simulink model "mod3_ciff_1bit"  (Simulink 7.9)
settings: Solver=ode45  StartTime=0.0  StopTime=simu.trantime  RelTol=1e-3
undefined symbols (not defined in the file): dc, Fs, mod, OSR, sinamp, sinfreq
libraries: dspsigops x3, dsparch4 x1, simulink x1, dspsrcs4 x1
settings Model: Creator=amyles  LastModifiedBy=Arnaldi Isacco
settings DataIOCC: LimitDataPoints=off  MaxDataPoints=50000
settings OptimizationCC: InlineParams=on
settings DebuggingCC: StrictBusMsg=Warning
settings ModelReferenceCC: ModelReferenceNumInstancesAllowed=Single
settings CodeAppCC: CustomSymbolStrType=$N$R$M_T
settings GRTTargetCC: CombineOutputUpdateFcns=off  GRTInterface=on

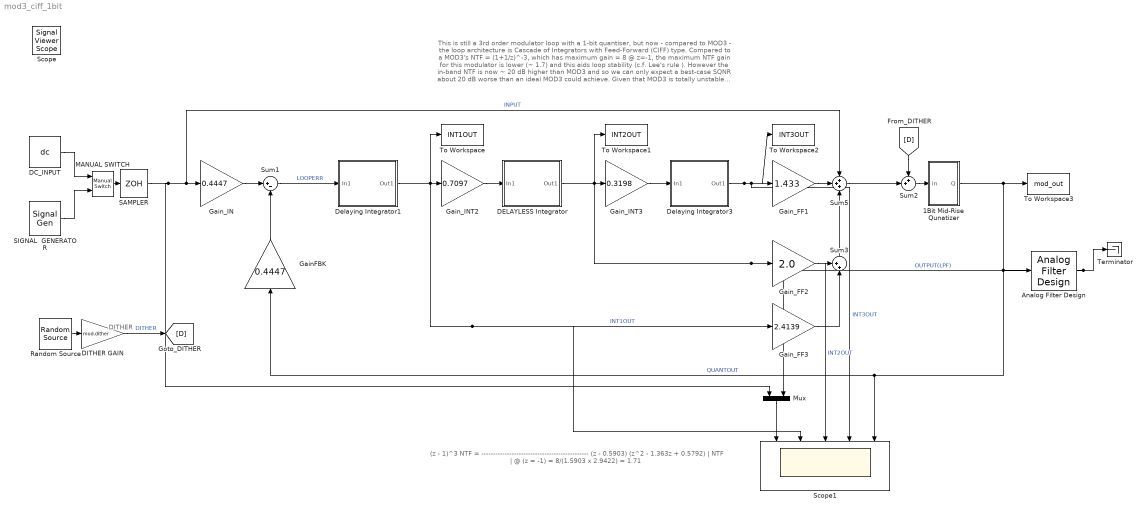
== system mod3_ciff_1bit ==
  note: This is still a 3rd order modulator loop with a 1-bit quantiser, but now - compared to MOD3 - the loop architecture is Cascade of Integrators
      | with Feed-Forward  (CIFF) type.  Compared to a MOD3's NTF = (1+1/z)^-3, which has maximum gain = 8 @ z=-1, the  maximum NTF gain for
      | this modulator is lower (~ 1.7) and this aids loop stability (c.f. Lee's rule ). However the in-band NTF is now ~ 20 dB higher than MOD3 and so
      | we can only expect a best-case SQNR about 20 dB worse than an ideal MOD3 could achieve.
      | Given that MOD3 is totally unstable and hence useless anyway, this still is a very acceptable cost to pay!
  note: (z - 1)^3
      |   NTF = ----------------------------------------------
      |            (z - 0.5903) (z^2 - 1.363z + 0.5792)
      |
      |
      | | NTF | @ (z = -1) = 8/(1.5903 x 2.9422) = 1.71
  note: DITHER
  1Bit Mid-Rise Qunatizer : Subsystem
  Analog Filter Design : dsparch4/Analog Filter Design  method=Butterworth  filttype=Lowpass  N=8  Wlo=pi*(Fs/OSR)  Whi=80  Rp=2  Rs=40
      settings: AttributesFormatString=Low-pass filter the loop output\nto illustrate intuitively how the\npulse density modulated +1/-1\noutput stream does indeed capture\nthe input signal
  DC_INPUT : Constant  Value=dc  VectorParams1D=off  OutDataTypeStr=double  SampleTime=1/Fs
  DELAYLESS Integrator : Subsystem
  DITHER GAIN : Gain  Gain=mod.dither  SampleTime=1/Fs
  Delaying Integrator1 : Subsystem
  Delaying Integrator3 : Subsystem
  GainFBK : Gain  Gain=0.4447
  Gain_FF1 : Gain  Gain=1.433
  Gain_FF2 : Gain  Gain=2.0
  Gain_FF3 : Gain  Gain=2.4139
  Gain_IN : Gain  Gain=0.4447
  Gain_INT2 : Gain  Gain=0.7097
  Gain_INT3 : Gain  Gain=0.3198
  MANUAL SWITCH : simulink/Signal Routing/Manual Switch  sw=0  action=0  varsize=off
      settings: AttributesFormatString=Double click to\nselect the desired\ninput
  Mux : Mux  Inputs=2
  Random Source : dspsrcs4/Random Source  SrcType=Uniform  NormMethod=Ziggurat  CltLength=12  MinVal=-1  MaxVal=1  MeanVal=0  VarVal=1  RepMode=Not repeatable  rawSeed=1  IsInherit=off  SampMode=Discrete  SampTime=1/Fs  SampFrame=1  DataType=Double  OutComplex=Real
  SAMPLER : ZeroOrderHold  SampleTime=1/Fs
  SIGNAL  GENERATOR : SignalGenerator  Amplitude=sinamp  Frequency=sinfreq  VectorParams1D=off
  Scope1 : Scope  NumInputPorts=5
      settings: TimeRange=2.089895171320487e-05  YMin=0.43~-0.6~-0.6~-0.3~-1.1  YMax=0.52~0.5~0.5~0.5~1.1
  Sum1 : Sum  Inputs=|+-  SampleTime=1/Fs
      settings: AttributesFormatString=Modulator input\nloop servo error (input - fbk)
  Sum2 : Sum  Inputs=++|
  Sum3 : Sum  Inputs=++|
  Sum5 : Sum  Inputs=+++
  Terminator : Terminator
  To Workspace : ToWorkspace  VariableName=INT1OUT  SampleTime=-1
  To Workspace1 : ToWorkspace  VariableName=INT2OUT  SampleTime=-1
  To Workspace2 : ToWorkspace  VariableName=INT3OUT  SampleTime=-1
  To Workspace3 : ToWorkspace  VariableName=mod_out  SampleTime=-1
      settings: AttributesFormatString=Export output to\nworkspace for\npost-processing
  Scope : SignalViewerScope  IOType=viewer  NumInputPorts=4  ZoomMode=xonly  RefreshTime=0.035000
      settings: YMin=-5~-5~-5~-5  YMax=5~5~5~5
  wires:
  Sum1/1 -> Delaying Integrator1/1(In1)  "LOOPERR"
  SAMPLER/1 -> Gain_IN/1, Sum5/1, Mux/1  "INPUT"
  1Bit Mid-Rise Qunatizer/1(Q) -> To Workspace3/1, Analog Filter Design/1, Scope1/5, GainFBK/1  "QUANTOUT"
  Delaying Integrator1/1(Out1) -> Gain_INT2/1, Gain_FF3/1, Scope1/2, To Workspace/1  "INT1OUT"
  Gain_INT2/1 -> DELAYLESS Integrator/1(In1)
  DELAYLESS Integrator/1(Out1) -> Gain_INT3/1, To Workspace1/1, Gain_FF2/1, Scope1/3  "INT2OUT"
  GainFBK/1 -> Sum1/2
  Gain_IN/1 -> Sum1/1
  Delaying Integrator3/1(Out1) -> Gain_FF1/1, To Workspace2/1, Scope1/4  "INT3OUT"
  Gain_INT3/1 -> Delaying Integrator3/1(In1)
  Gain_FF1/1 -> Sum5/2
  Gain_FF2/1 -> Sum3/1
  Sum3/1 -> Sum5/3
  Gain_FF3/1 -> Sum3/2
  Random Source/1 -> DITHER GAIN/1
  DITHER GAIN/1 -> [D]  "DITHER"
  [D] -> Sum2/1
  Sum2/1 -> 1Bit Mid-Rise Qunatizer/1(in)
  Sum5/1 -> Sum2/2
  Analog Filter Design/1 -> Terminator/1, Mux/2  "OUTPUT(LPF)"
  DC_INPUT/1 -> MANUAL SWITCH/1
  SIGNAL  GENERATOR/1 -> MANUAL SWITCH/2
  MANUAL SWITCH/1 -> SAMPLER/1
  Mux/1 -> Scope1/1

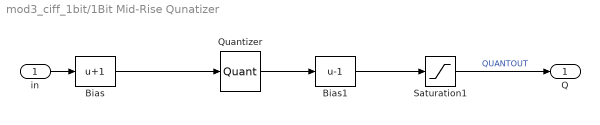
== system mod3_ciff_1bit/1Bit Mid-Rise Qunatizer ==
  in : Inport
  Bias : Bias  Bias=1
      settings: AttributesFormatString=Need offset to give\nMID-RISE quantiser
  Bias1 : Bias  Bias=-1
  Quantizer : Quantizer  QuantizationInterval=2  LinearizeAsGain=off  SampleTime=1/Fs
  Saturation1 : Saturate  UpperLimit=1  LowerLimit=-1
      settings: AttributesFormatString=Limit quantiser\noutput to +/-1
  Q : Outport
  wires:
  Bias/1 -> Quantizer/1
  Quantizer/1 -> Bias1/1
  Bias1/1 -> Saturation1/1
  in/1 -> Bias/1
  Saturation1/1 -> Q/1  "QUANTOUT"

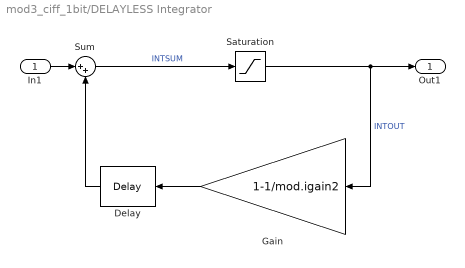
== system mod3_ciff_1bit/DELAYLESS Integrator ==
  In1 : Inport
  Delay : dspsigops/Delay  InputProcessing=Inherited (this choice will be removed - see release notes)  dly_unit=Samples  delay=1  ic_detail=off  dif_ic_for_ch=off  dif_ic_for_dly=off  ic=0  reset_popup=None
  Gain : Gain  Gain=1-1/mod.igain2
      settings: AttributesFormatString=Integrator leakage
  Saturation : Saturate  UpperLimit=mod.isat2  LowerLimit=-(mod.isat2)
  Sum : Sum  Inputs=|++
      settings: AttributesFormatString=Integrator summer
  Out1 : Outport
  wires:
  In1/1 -> Sum/1
  Saturation/1 -> Out1/1, Gain/1  "INTOUT"
  Gain/1 -> Delay/1
  Sum/1 -> Saturation/1  "INTSUM"
  Delay/1 -> Sum/2

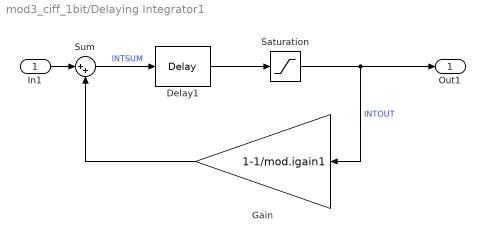
== system mod3_ciff_1bit/Delaying Integrator1 ==
  In1 : Inport
  Delay1 : dspsigops/Delay  InputProcessing=Inherited (this choice will be removed - see release notes)  dly_unit=Samples  delay=1  ic_detail=off  dif_ic_for_ch=off  dif_ic_for_dly=off  ic=0  reset_popup=None
  Gain : Gain  Gain=1-1/mod.igain1
      settings: AttributesFormatString=Integrator leakage
  Saturation : Saturate  UpperLimit=mod.isat1  LowerLimit=-(mod.isat1)
  Sum : Sum  Inputs=|++
      settings: AttributesFormatString=Integrator summer
  Out1 : Outport
  wires:
  Sum/1 -> Delay1/1  "INTSUM"
  Gain/1 -> Sum/2
  Saturation/1 -> Gain/1, Out1/1  "INTOUT"
  In1/1 -> Sum/1
  Delay1/1 -> Saturation/1

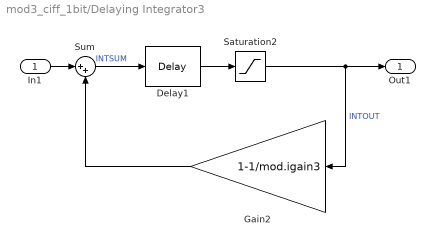
== system mod3_ciff_1bit/Delaying Integrator3 ==
  In1 : Inport
  Delay1 : dspsigops/Delay  InputProcessing=Inherited (this choice will be removed - see release notes)  dly_unit=Samples  delay=1  ic_detail=off  dif_ic_for_ch=off  dif_ic_for_dly=off  ic=0  reset_popup=None
  Gain2 : Gain  Gain=1-1/mod.igain3
      settings: AttributesFormatString=Integrator leakage
  Saturation2 : Saturate  UpperLimit=mod.isat3  LowerLimit=-(mod.isat3)
  Sum : Sum  Inputs=|++
      settings: AttributesFormatString=Integrator summer
  Out1 : Outport
  wires:
  Sum/1 -> Delay1/1  "INTSUM"
  Gain2/1 -> Sum/2
  Saturation2/1 -> Gain2/1, Out1/1  "INTOUT"
  In1/1 -> Sum/1
  Delay1/1 -> Saturation2/1
